simulink model "System_Modell"  (R2017b)
settings: Solver=VariableStepAuto  StartTime=0.0  StopTime=10  RelTol=1e-3
settings Model: Creator=张紫薇  LastModifiedBy=张紫薇

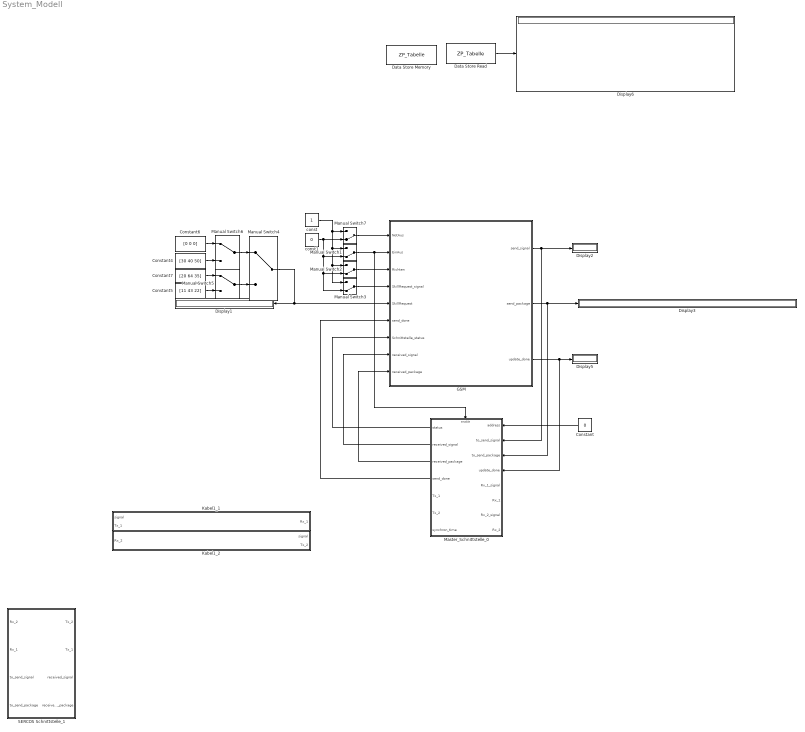
== system System_Modell ==
  Constant : Constant  Value=0
  Constant4 : Constant  Value=[30 40 50]
  Constant5 : Constant  Value=[11 43 22]
  Constant6 : Constant  Value=[0 0 0]
  Constant7 : Constant  Value=[20 64 35]
  Data Store Memory : DataStoreMemory  DataStoreName=ZP_Tabelle  ReadBeforeWriteMsg=warning  WriteAfterWriteMsg=warning  WriteAfterReadMsg=warning  InitialValue=zeros(10,7)  ShowAdditionalParam=off  OutDataTypeStr=double  Dimensions=[10 7]
  Data Store Read : DataStoreRead  DataStoreName=ZP_Tabelle
  Display{1..3,5..6} (5 alike) : Display
  "GSM " : Subsystem
  Kabel1_1 : Subsystem
  Kabel1_2 : Subsystem
  Manual Switch{1..3,7} (4 alike) : ManualSwitch  CurrentSetting=0
  Manual Switch4 : ManualSwitch
  Manual Switch5 : ManualSwitch
  Manual Switch6 : ManualSwitch
  Master_Schnittstelle_0 : Subsystem
  SERCOS Schnittstelle_1 : Subsystem
  const : Constant  OutDataTypeStr=boolean
  const1 : Constant  Value=0  OutDataTypeStr=boolean
  wires:
  Manual Switch6/1 -> Manual Switch4/1
  Constant5/1 -> Manual Switch5/2
  Manual Switch5/1 -> Manual Switch4/2
  Manual Switch3/1 -> "GSM "/4(SkillRequest_signal)
  Data Store Read/1 -> Display6/1
  Constant7/1 -> Manual Switch5/1
  const1/1 -> Manual Switch2/2, Manual Switch3/2, Manual Switch1/2, Manual Switch7/2
  "GSM "/2(send_package) -> Display3/1, Master_Schnittstelle_0/3(to_send_package)
  "GSM "/3(update_done) -> Master_Schnittstelle_0/4(update_done), Display5/1
  const/1 -> Manual Switch3/1, Manual Switch2/1, Manual Switch1/1, Manual Switch7/1
  Manual Switch7/1 -> "GSM "/1(NotAus)
  Constant6/1 -> Manual Switch6/1
  Manual Switch2/1 -> "GSM "/3(Richten)
  Manual Switch1/1 -> Master_Schnittstelle_0/Enable, "GSM "/2(EinAus)
  Manual Switch4/1 -> "GSM "/5(SkillRequest), Display1/1
  "GSM "/1(send_signal) -> Display2/1, Master_Schnittstelle_0/2(to_send_signal)
  Constant4/1 -> Manual Switch6/2
  Master_Schnittstelle_0/1(status) -> "GSM "/7(Schnittstelle_status)
  Master_Schnittstelle_0/4(send_done) -> "GSM "/6(send_done)
  Master_Schnittstelle_0/2(received_signal) -> "GSM "/8(received_signal)
  Master_Schnittstelle_0/3(received_package) -> "GSM "/9(received_package)
  Constant/1 -> Master_Schnittstelle_0/1(address)

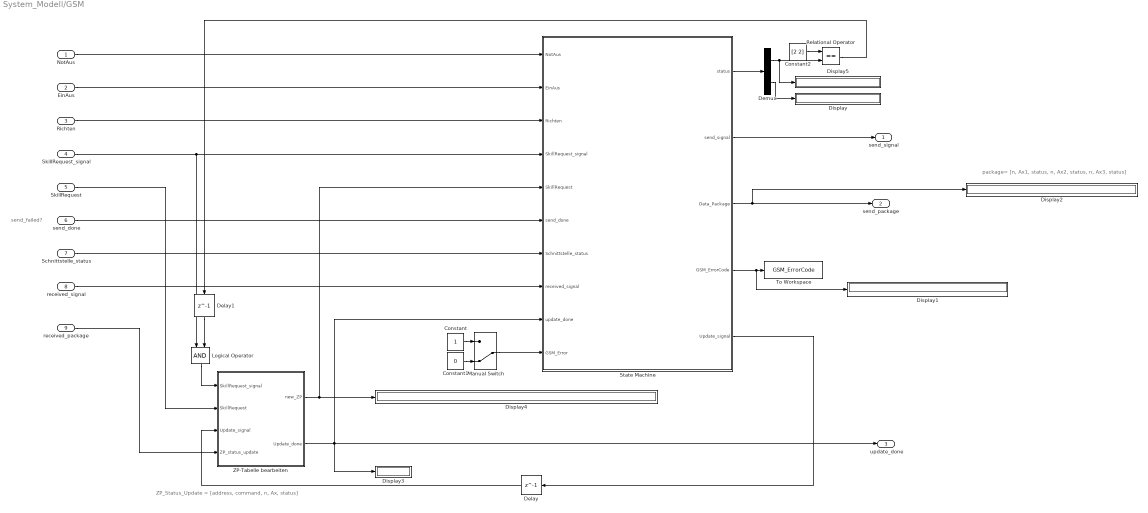
== system System_Modell/GSM  ==
  note: send_failed?
  note: package= [n, Ax1, status, n, Ax2, status, n, Ax3, status]
  note: ZP_Status_Update = [address, command, n, Ax, status]
  NotAus : Inport  OutDataTypeStr=boolean
  EinAus : Inport  Port=2  OutDataTypeStr=boolean
  Richten : Inport  Port=3  OutDataTypeStr=boolean
  SkillRequest_signal : Inport  Port=4  OutDataTypeStr=boolean
  SkillRequest : Inport  Port=5  OutDataTypeStr=double  PortDimensions=3
  send_done : Inport  Port=6  OutDataTypeStr=boolean
  Schnittstelle_status : Inport  Port=7  OutDataTypeStr=double
  received_signal : Inport  Port=8  OutDataTypeStr=boolean
  received_package : Inport  Port=9  OutDataTypeStr=double  PortDimensions=5
  Constant : Constant  OutDataTypeStr=boolean
  Constant1 : Constant  Value=0  OutDataTypeStr=boolean
  Constant2 : Constant  Value=[2 2]  OutDataTypeStr=double
  Delay : Delay  DelayLength=1
  Delay1 : Delay  DelayLength=1
  Demux : Demux  Outputs=2
  Display{,1..5} (6 alike) : Display
  Logical Operator : Logic  AllPortsSameDT=off  OutDataTypeStr=boolean
  Manual Switch : ManualSwitch  CurrentSetting=0
  Relational Operator : RelationalOperator  Operator===  OutDataTypeStr=boolean  RndMeth=Simplest
  State Machine : Stateflow chart  TreatAsAtomicUnit=on
  To Workspace : ToWorkspace  VariableName=GSM_ErrorCode  SaveFormat=Timeseries  SampleTime=-1
  ZP-Tabelle bearbeiten : Subsystem
  send_signal : Outport  OutDataTypeStr=boolean
  send_package : Outport  Port=2  OutDataTypeStr=double  PortDimensions=7
  update_done : Outport  Port=3
  wires:
  received_signal/1 -> State Machine/8(received_signal)
  Richten/1 -> State Machine/3(Richten)
  NotAus/1 -> State Machine/1(NotAus)
  EinAus/1 -> State Machine/2(EinAus)
  Schnittstelle_status/1 -> State Machine/7(Schnittstelle_status)
  State Machine/4(GSM_ErrorCode) -> Display1/1, To Workspace/1
  SkillRequest_signal/1 -> State Machine/4(SkillRequest_signal), Logical Operator/1
  SkillRequest/1 -> ZP-Tabelle bearbeiten/2(SkillRequest)
  Constant/1 -> Manual Switch/1
  Constant1/1 -> Manual Switch/2
  Manual Switch/1 -> State Machine/10(GSM_Error)
  State Machine/2(send_signal) -> send_signal/1
  State Machine/3(Data_Package) -> Display2/1, send_package/1
  received_package/1 -> ZP-Tabelle bearbeiten/4(ZP_status_update)
  ZP-Tabelle bearbeiten/1(new_ZP) -> State Machine/5(SkillRequest), Display4/1
  send_done/1 -> State Machine/6(send_done)
  ZP-Tabelle bearbeiten/2(Update_done) -> update_done/1, State Machine/9(update_done), Display3/1
  State Machine/5(Update_signal) -> Delay/1
  Delay/1 -> ZP-Tabelle bearbeiten/3(Update_signal)
  Demux/2 -> Display/1
  State Machine/1(status) -> Demux/1
  Constant2/1 -> Relational Operator/1
  Demux/1 -> Display5/1, Relational Operator/2
  Relational Operator/1 -> Delay1/1
  Delay1/1 -> Logical Operator/2
  Logical Operator/1 -> ZP-Tabelle bearbeiten/1(SkillRequest_signal)

== system System_Modell/Kabel1_1 ==
  Rx_1 : Inport
  Delay : Delay  DelayLength=1
  signal : Outport
  Tx_1 : Outport  Port=2
  wires:
  Rx_1/1 -> Delay/1, Tx_1/1
  Delay/1 -> signal/1

== system System_Modell/Kabel1_2 ==
  Rx_2 : Inport
  Delay : Delay  DelayLength=1
  signal : Outport
  Tx_2 : Outport  Port=2
  wires:
  Rx_2/1 -> Delay/1, Tx_2/1
  Delay/1 -> signal/1

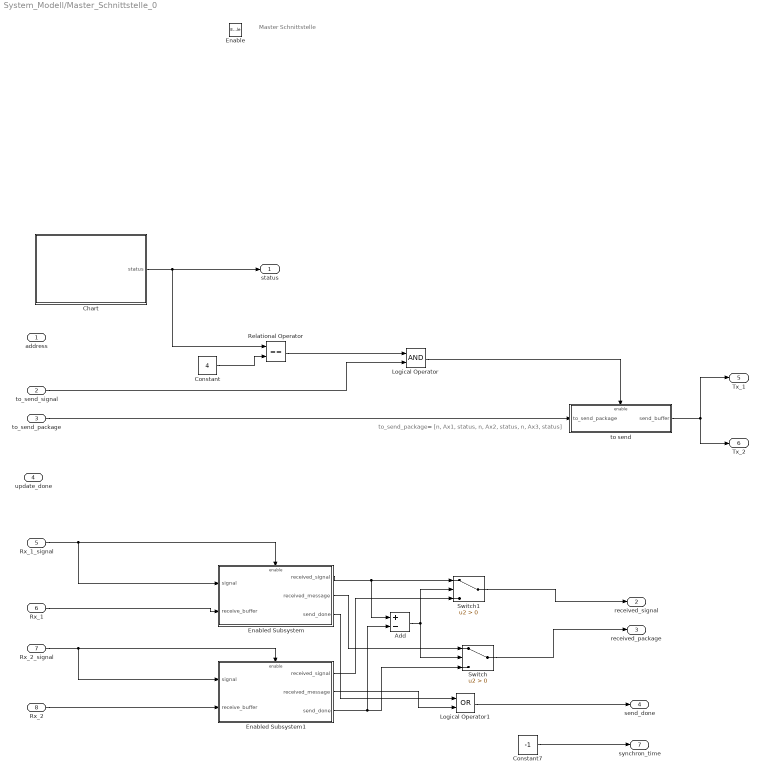
== system System_Modell/Master_Schnittstelle_0 ==
  note: Master Schnittstelle
  note: to_send_package= [n, Ax1, status, n, Ax2, status, n, Ax3, status]
  address : Inport
  to_send_signal : Inport  Port=2
  to_send_package : Inport  Port=3
  update_done : Inport  Port=4
  Rx_1_signal : Inport  Port=5
  Rx_1 : Inport  Port=6
  Rx_2_signal : Inport  Port=7
  Rx_2 : Inport  Port=8
  Enable : EnablePort
  Add : Sum  Inputs=+-
  Chart : Stateflow chart  TreatAsAtomicUnit=on
  Constant : Constant  Value=4
  Constant7 : Constant  Value=-1
  Enabled Subsystem : Subsystem  TreatAsAtomicUnit=on
  Enabled Subsystem1 : Subsystem  TreatAsAtomicUnit=on
  Logical Operator : Logic  AllPortsSameDT=off  OutDataTypeStr=boolean
  Logical Operator1 : Logic  Operator=OR  AllPortsSameDT=off  OutDataTypeStr=boolean
  Relational Operator : RelationalOperator  Operator===  OutDataTypeStr=boolean  RndMeth=Simplest
  Switch : Switch  Criteria=u2 > Threshold
  Switch1 : Switch  Criteria=u2 > Threshold
  to send : Subsystem  TreatAsAtomicUnit=on
  status : Outport
  received_signal : Outport  Port=2
  received_package : Outport  Port=3
  send_done : Outport  Port=4
  Tx_1 : Outport  Port=5
  Tx_2 : Outport  Port=6
  synchron_time : Outport  Port=7
  wires:
  Constant/1 -> Relational Operator/2
  Relational Operator/1 -> Logical Operator/1
  to_send_signal/1 -> Logical Operator/2
  Logical Operator/1 -> to send/Enable
  to_send_package/1 -> to send/1(to_send_package)
  Rx_1/1 -> Enabled Subsystem/2(receive_buffer)
  Chart/1(status) -> status/1, Relational Operator/1
  Rx_1_signal/1 -> Enabled Subsystem/Enable, Enabled Subsystem/1(signal)
  Rx_2_signal/1 -> Enabled Subsystem1/Enable, Enabled Subsystem1/1(signal)
  Rx_2/1 -> Enabled Subsystem1/2(receive_buffer)
  Enabled Subsystem/2(received_message) -> Switch/1
  Enabled Subsystem1/3(send_done) -> Add/2, Switch/3
  Switch/1 -> received_package/1
  Enabled Subsystem/1(received_signal) -> Add/1, Switch1/1
  Enabled Subsystem1/1(received_signal) -> Switch1/3
  Switch1/1 -> received_signal/1
  Add/1 -> Switch1/2, Switch/2
  to send/1(send_buffer) -> Tx_2/1, Tx_1/1
  Enabled Subsystem/3(send_done) -> Logical Operator1/1
  Enabled Subsystem1/2(received_message) -> Logical Operator1/2
  Logical Operator1/1 -> send_done/1
  Constant7/1 -> synchron_time/1

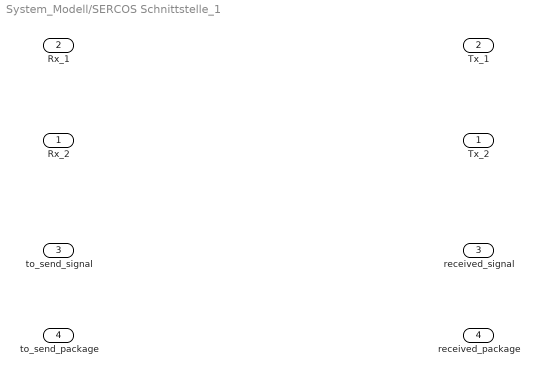
== system System_Modell/SERCOS Schnittstelle_1 ==
  Rx_2 : Inport
  Rx_1 : Inport  Port=2
  to_send_signal : Inport  Port=3
  to_send_package : Inport  Port=4
  Tx_2 : Outport
  Tx_1 : Outport  Port=2
  received_signal : Outport  Port=3
  received_package : Outport  Port=4

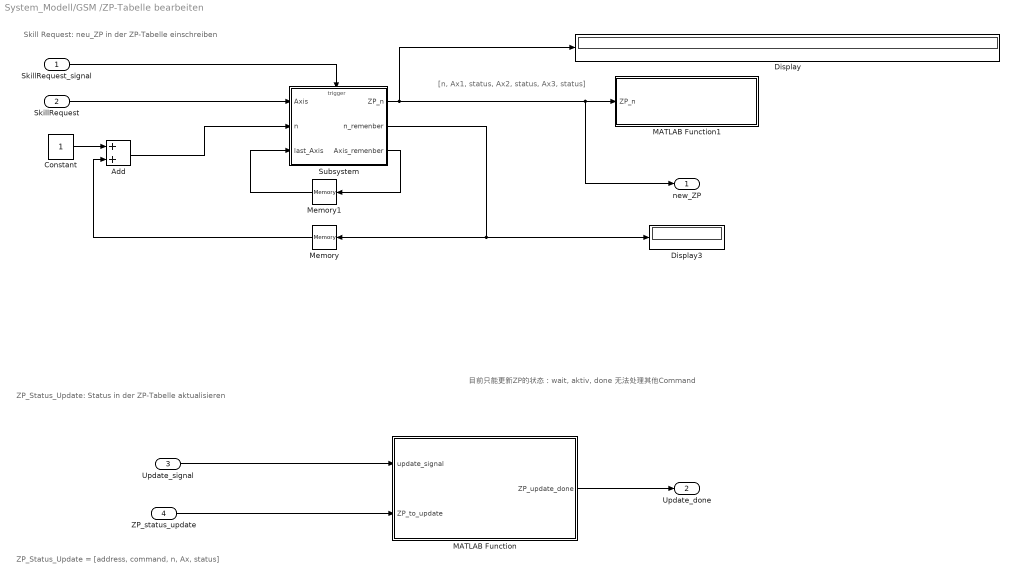
== system System_Modell/GSM /ZP-Tabelle bearbeiten ==
  note: ZP_Status_Update = [address, command, n, Ax, status]
  note: Skill Request: neu_ZP in der ZP-Tabelle einschreiben
  note: ZP_Status_Update: Status in der ZP-Tabelle aktualisieren
  note: [n, Ax1, status, Ax2, status, Ax3, status]
  note: 目前只能更新ZP的状态：wait, aktiv, done
      | 无法处理其他Command
  SkillRequest_signal : Inport  OutDataTypeStr=boolean
  SkillRequest : Inport  Port=2  OutDataTypeStr=double  PortDimensions=3
  Update_signal : Inport  Port=3  OutDataTypeStr=boolean
  ZP_status_update : Inport  Port=4  OutDataTypeStr=double  PortDimensions=5
  Add : Sum
  Constant : Constant
  Display : Display
  Display3 : Display
  MATLAB Function : MATLAB Function  TreatAsAtomicUnit=on
  MATLAB Function1 : MATLAB Function  TreatAsAtomicUnit=on
  Memory : Memory
  Memory1 : Memory  InitialCondition=[0 0 0]
  Subsystem : Subsystem
  new_ZP : Outport
  Update_done : Outport  Port=2  OutDataTypeStr=boolean
  wires:
  Memory1/1 -> Subsystem/3(last_Axis)
  Subsystem/3(Axis_remenber) -> Memory1/1
  SkillRequest/1 -> Subsystem/1(Axis)
  Update_signal/1 -> MATLAB Function/1(update_signal)
  Add/1 -> Subsystem/2(n)
  ZP_status_update/1 -> MATLAB Function/2(ZP_to_update)
  MATLAB Function/1(ZP_update_done) -> Update_done/1
  Constant/1 -> Add/1
  SkillRequest_signal/1 -> Subsystem/Trigger
  Memory/1 -> Add/2
  Subsystem/2(n_remenber) -> Memory/1, Display3/1
  Subsystem/1(ZP_n) -> Display/1, MATLAB Function1/1(ZP_n), new_ZP/1

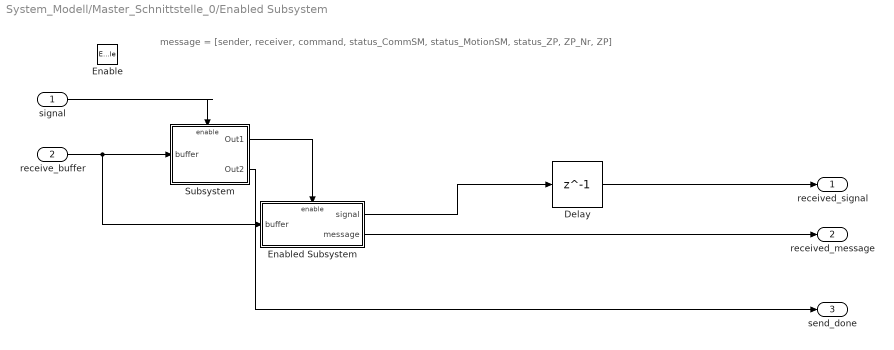
== system System_Modell/Master_Schnittstelle_0/Enabled Subsystem ==
  note: message = [sender, receiver, command, status_CommSM, status_MotionSM, status_ZP, ZP_Nr, ZP]
  signal : Inport
  receive_buffer : Inport  Port=2
  Enable : EnablePort
  Delay : Delay  DelayLength=1
  Enabled Subsystem : Subsystem  TreatAsAtomicUnit=on
  Subsystem : Subsystem
  received_signal : Outport
  received_message : Outport  Port=2
  send_done : Outport  Port=3
  wires:
  receive_buffer/1 -> Enabled Subsystem/1(buffer), Subsystem/1(buffer)
  Subsystem/1(Out1) -> Enabled Subsystem/Enable
  signal/1 -> Subsystem/Enable
  Enabled Subsystem/2(message) -> received_message/1
  Enabled Subsystem/1(signal) -> Delay/1
  Delay/1 -> received_signal/1
  Subsystem/2(Out2) -> send_done/1

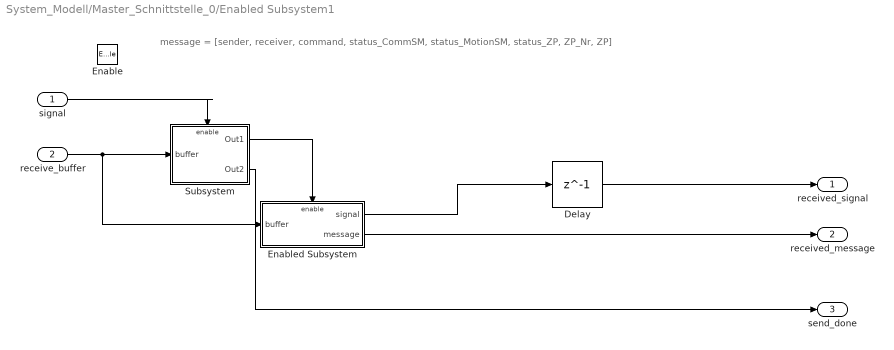
== system System_Modell/Master_Schnittstelle_0/Enabled Subsystem1 ==
  note: message = [sender, receiver, command, status_CommSM, status_MotionSM, status_ZP, ZP_Nr, ZP]
  signal : Inport
  receive_buffer : Inport  Port=2
  Enable : EnablePort
  Delay : Delay  DelayLength=1
  Enabled Subsystem : Subsystem  TreatAsAtomicUnit=on
  Subsystem : Subsystem
  received_signal : Outport
  received_message : Outport  Port=2
  send_done : Outport  Port=3
  wires:
  receive_buffer/1 -> Enabled Subsystem/1(buffer), Subsystem/1(buffer)
  Subsystem/1(Out1) -> Enabled Subsystem/Enable
  signal/1 -> Subsystem/Enable
  Enabled Subsystem/2(message) -> received_message/1
  Enabled Subsystem/1(signal) -> Delay/1
  Delay/1 -> received_signal/1
  Subsystem/2(Out2) -> send_done/1

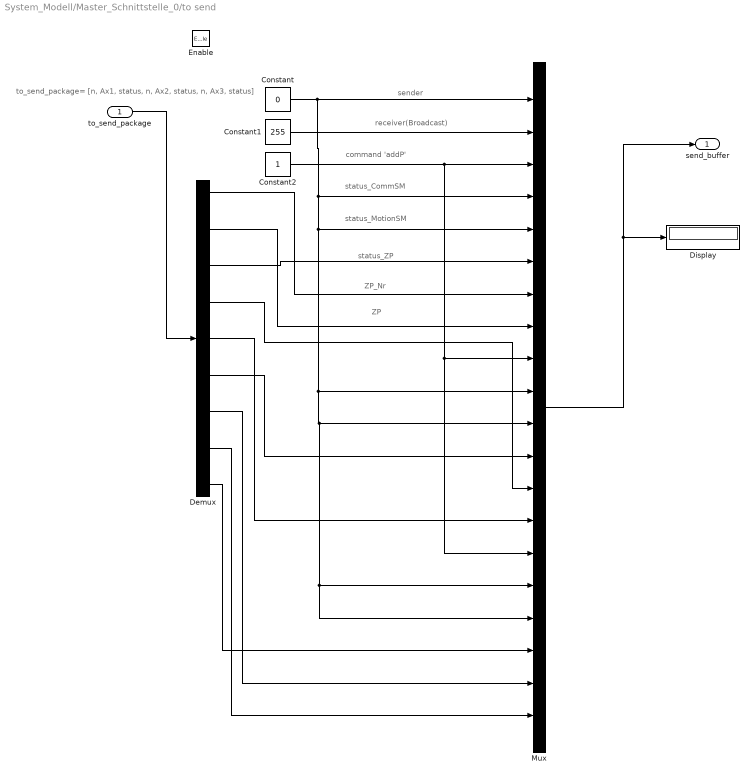
== system System_Modell/Master_Schnittstelle_0/to send ==
  note: ZP
  note: ZP_Nr
  note: status_ZP
  note: status_MotionSM
  note: status_CommSM
  note: command 'addP'
  note: receiver(Broadcast)
  note: sender
  note: to_send_package= [n, Ax1, status, n, Ax2, status, n, Ax3, status]
  to_send_package : Inport
  Enable : EnablePort
  Constant : Constant  Value=0
  Constant1 : Constant  Value=255
  Constant2 : Constant
  Demux : Demux  Outputs=9
  Display : Display
  Mux : Mux  Inputs=20
  send_buffer : Outport
  wires:
  to_send_package/1 -> Demux/1
  Constant/1 -> Mux/1, Mux/5, Mux/10, Mux/16, Mux/17, Mux/11, Mux/4
  Constant1/1 -> Mux/2
  Constant2/1 -> Mux/15, Mux/9, Mux/3
  Demux/3 -> Mux/6
  Demux/1 -> Mux/7
  Demux/2 -> Mux/8
  Demux/6 -> Mux/12
  Demux/4 -> Mux/13
  Demux/5 -> Mux/14
  Demux/9 -> Mux/18
  Demux/7 -> Mux/19
  Demux/8 -> Mux/20
  Mux/1 -> Display/1, send_buffer/1

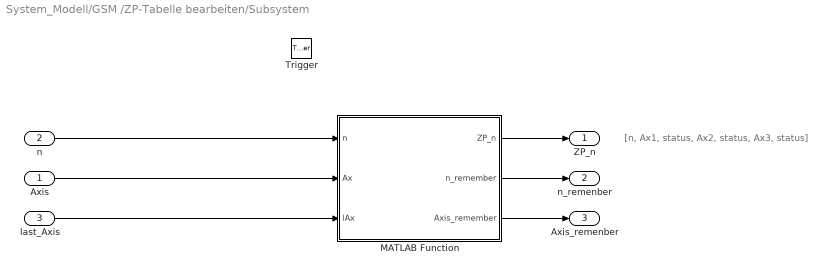
== system System_Modell/GSM /ZP-Tabelle bearbeiten/Subsystem ==
  note: [n, Ax1, status, Ax2, status, Ax3, status]
  Axis : Inport
  n : Inport  Port=2
  last_Axis : Inport  Port=3
  Trigger : TriggerPort  VariantControl=Variant  PortDimensions=1
  MATLAB Function : MATLAB Function  TreatAsAtomicUnit=on
  ZP_n : Outport
  n_remenber : Outport  Port=2
  Axis_remenber : Outport  Port=3
  wires:
  n/1 -> MATLAB Function/1(n)
  Axis/1 -> MATLAB Function/2(Ax)
  MATLAB Function/1(ZP_n) -> ZP_n/1
  last_Axis/1 -> MATLAB Function/3(lAx)
  MATLAB Function/2(n_remember) -> n_remenber/1
  MATLAB Function/3(Axis_remember) -> Axis_remenber/1

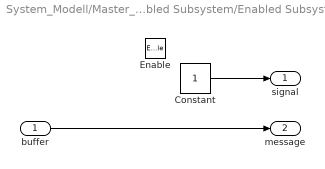
== system System_Modell/Master_Schnittstelle_0/Enabled Subsystem/Enabled Subsystem ==
  buffer : Inport
  Enable : EnablePort
  Constant : Constant
  signal : Outport
  message : Outport  Port=2
  wires:
  buffer/1 -> message/1
  Constant/1 -> signal/1

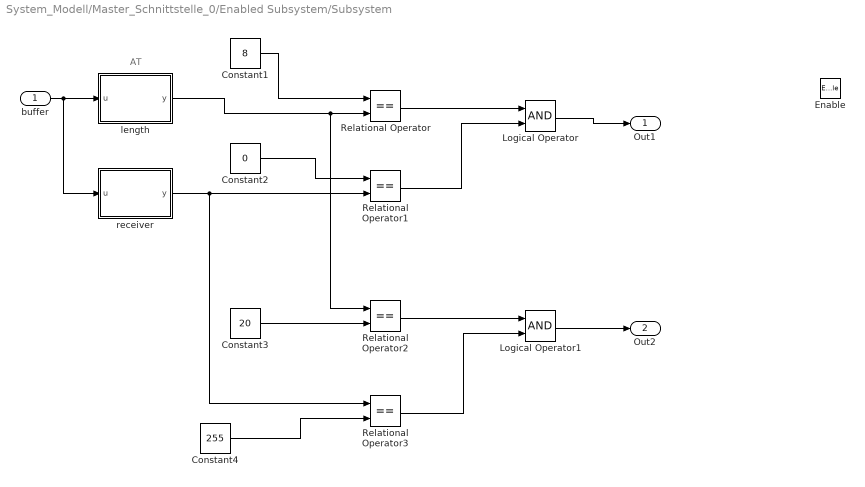
== system System_Modell/Master_Schnittstelle_0/Enabled Subsystem/Subsystem ==
  note: AT
  buffer : Inport
  Enable : EnablePort
  Constant1 : Constant  Value=8
  Constant2 : Constant  Value=0
  Constant3 : Constant  Value=20
  Constant4 : Constant  Value=255
  Logical Operator : Logic  AllPortsSameDT=off  OutDataTypeStr=boolean
  Logical Operator1 : Logic  AllPortsSameDT=off  OutDataTypeStr=boolean
  Relational Operator{,1..3} (4 alike) : RelationalOperator  Operator===  OutDataTypeStr=boolean  RndMeth=Simplest
  length : MATLAB Function  TreatAsAtomicUnit=on
  receiver : MATLAB Function  TreatAsAtomicUnit=on
  Out1 : Outport
  Out2 : Outport  Port=2
  wires:
  Constant2/1 -> Relational Operator1/1
  buffer/1 -> receiver/1(u), length/1(u)
  length/1(y) -> Relational Operator2/1, Relational Operator/2
  Constant1/1 -> Relational Operator/1
  receiver/1(y) -> Relational Operator3/1, Relational Operator1/2
  Relational Operator/1 -> Logical Operator/1
  Relational Operator1/1 -> Logical Operator/2
  Logical Operator/1 -> Out1/1
  Constant3/1 -> Relational Operator2/2
  Relational Operator2/1 -> Logical Operator1/1
  Constant4/1 -> Relational Operator3/2
  Relational Operator3/1 -> Logical Operator1/2
  Logical Operator1/1 -> Out2/1

== system System_Modell/Master_Schnittstelle_0/Enabled Subsystem1/Enabled Subsystem ==
  buffer : Inport
  Enable : EnablePort
  Constant : Constant
  signal : Outport
  message : Outport  Port=2
  wires:
  buffer/1 -> message/1
  Constant/1 -> signal/1

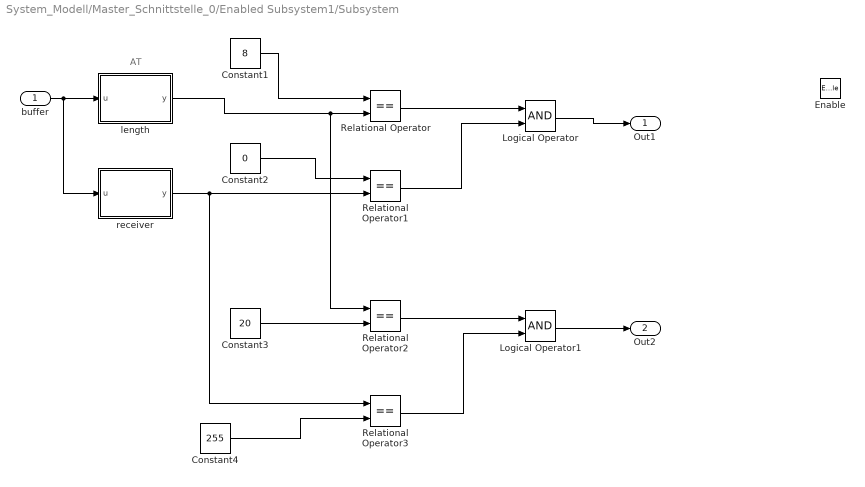
== system System_Modell/Master_Schnittstelle_0/Enabled Subsystem1/Subsystem ==
  note: AT
  buffer : Inport
  Enable : EnablePort
  Constant1 : Constant  Value=8
  Constant2 : Constant  Value=0
  Constant3 : Constant  Value=20
  Constant4 : Constant  Value=255
  Logical Operator : Logic  AllPortsSameDT=off  OutDataTypeStr=boolean
  Logical Operator1 : Logic  AllPortsSameDT=off  OutDataTypeStr=boolean
  Relational Operator{,1..3} (4 alike) : RelationalOperator  Operator===  OutDataTypeStr=boolean  RndMeth=Simplest
  length : MATLAB Function  TreatAsAtomicUnit=on
  receiver : MATLAB Function  TreatAsAtomicUnit=on
  Out1 : Outport
  Out2 : Outport  Port=2
  wires:
  Constant2/1 -> Relational Operator1/1
  buffer/1 -> receiver/1(u), length/1(u)
  length/1(y) -> Relational Operator2/1, Relational Operator/2
  Constant1/1 -> Relational Operator/1
  receiver/1(y) -> Relational Operator3/1, Relational Operator1/2
  Relational Operator/1 -> Logical Operator/1
  Relational Operator1/1 -> Logical Operator/2
  Logical Operator/1 -> Out1/1
  Constant3/1 -> Relational Operator2/2
  Relational Operator2/1 -> Logical Operator1/1
  Constant4/1 -> Relational Operator3/2
  Relational Operator3/1 -> Logical Operator1/2
  Logical Operator1/1 -> Out2/1

== stateflow chart System_Modell/GSM /State Machine ==
  settings: executeAtInitialization=1
  state NotAus
    entry: status=[1 0 0 0]
  state Aus
    entry: status=[0 0 0 0]
  state Ein
    entry: status=[2 0 0 0]
    note: status_Schnittstelle: CP0 - CP4
    state Init
      entry: status=[2 1 0 0]
    state Error
      entry: status=[2 3 0 0];
    state Run
      entry: status= [2 2 0 0]
      state Stand_By
        entry: status = [2 2 1 0];
      state Send_ZP
        entry: status = [2 2 2 0]; send_signal=SkillRequest_signal; Data_Package = SkillRequest
      note: wann send_signal=0 ???
      state ZP_Status_Update
        entry: status = [2 2 3 0]; Update_signal = received_signal
      note: ZP_Status_Update = [address, command, n, Ax, status]
      note: received_package = [address, command, n, Ax, status]
      (default) -> Stand_By
      Stand_By -> Send_ZP [order 1] : [SkillRequest_signal && ~send_done]
      Send_ZP -> Stand_By : [send_done && ~SkillRequest_signal]{send_signal=false;}
      ZP_Status_Update -> Stand_By : [update_done && ~received_signal]{Update_signal=false;}
      Stand_By -> ZP_Status_Update [order 2] : [received_signal && ~update_done]
    Error -> Init : [GSM_Error==0] {GSM_ErrorCode=[0 0  0 0]}
    (default) -> Init
    Init -> Error [order 2] : [GSM_Error]{GSM_ErrorCode=status}
    Run -> Error [order 1] : [GSM_Error]{GSM_ErrorCode=status}
    Run -> Init [order 2] : [Schnittstelle_status~=4 && GSM_Error==0]
    Init -> Run [order 1] : [Schnittstelle_status==4]
  NotAus -> Aus [order 2] : [EinAus==0]
  Aus -> NotAus [order 1] : [EinAus==1 && NotAus==1]
  (default) -> Aus
  Ein -> NotAus [order 2] : [NotAus==1]
  NotAus -> Ein [order 1] : [NotAus==0 && Richten==1]
  Ein -> Aus [order 1] : [EinAus==0]
  Aus -> Ein [order 2] : [EinAus==1 && NotAus==0]
  data: NotAus input boolean; EinAus input boolean; Richten input boolean; SkillRequest_signal input boolean; SkillRequest input double size=7; send_done input boolean; Schnittstelle_status input double; status output double; send_signal output boolean; received_signal input boolean; update_done input boolean; GSM_Error input boolean; Data_Package output double size=7; GSM_ErrorCode output double; Update_signal output boolean size=1

== matlab function System_Modell/GSM /ZP-Tabelle bearbeiten/MATLAB Function ==
  data: update_signal input boolean; ZP_to_update input double size=5; ZP_update_done output boolean; ZP_Tabelle data_store_memory
%ZP_Status_Update = [address, command, n, Ax, status]
%function [ZP_update_done, Update_Data] = Status_Update(update_signal, ZP_to_update, ZP_Tab)

function ZP_update_done  = Status_Update(update_signal, ZP_to_update)

global ZP_Tabelle

N=0;
m=0;
n=0;

if update_signal == true
    address = ZP_to_update(1);
    m = 2 * address + 1;
    n = ZP_to_update(3);
    status = ZP_to_update(5);
    
    for i=1:10
        if ZP_Tabelle(i,1) == n
            N = i;              %ZP_N bestimmen
            break
        end
    end
    
    %N==1, status aktualisieren
    %N>1 && (status von ZP_N-1 == 'done'), status aktualisieren
    if (N == 1) || (N>1 && (ZP_Tabelle(N-1,3) == ZP_Tabelle(N-1,5) == ZP_Tabelle(N-1,7) == 3))
        ZP_Tabelle(N,m) = status;
        ZP_update_done = true;
    else        
        ZP_update_done = false;
    end
else
    ZP_update_done = false;
end

%Update_Data = ZP_Tabelle;

== stateflow chart System_Modell/Master_Schnittstelle_0/Chart ==
  state Start
    entry: status=-2
  state CP1
    entry: status=1
  state NRT
    entry: status=-1
  state CP0
    entry: status=0
  state CP2
    entry: status=2
  state CP3
    entry: status=3
  state CP4
    entry: status=4
  (default) -> Start
  CP0 -> CP1 [order 1]
  CP1 -> CP0 [order 2]
  Start -> NRT
  CP1 -> CP2 [order 1]
  CP2 -> CP0 [order 2]
  NRT -> CP0
  CP0 -> NRT [order 2]
  CP2 -> CP3 [order 1]
  CP4 -> CP0
  CP3 -> CP0 [order 2]
  CP3 -> CP4 [order 1]
  data: status output

== matlab function System_Modell/Master_Schnittstelle_0/Enabled Subsystem/Subsystem/length ==
  data: u input; y output
function y = fcn(u)

y = length(u);

== matlab function System_Modell/Master_Schnittstelle_0/Enabled Subsystem/Subsystem/receiver ==
  data: u input; y output
function y = fcn(u)

y = u(2);

== matlab function System_Modell/Master_Schnittstelle_0/Enabled Subsystem1/Subsystem/length ==
  data: u input; y output
function y = fcn(u)

y = length(u);

== matlab function System_Modell/Master_Schnittstelle_0/Enabled Subsystem1/Subsystem/receiver ==
  data: u input; y output
function y = fcn(u)

y = u(2);

== matlab function System_Modell/GSM /ZP-Tabelle bearbeiten/MATLAB Function1 ==
  data: ZP_n input; ZP_Tabelle data_store_memory
%ZP_n = [n, Ax1, status1, Ax2, status2, Ax3, status3];
%function ZP_newTable = new_ZP(ZP_n)

function new_ZP(ZP_n)

global ZP_Tabelle

m=0;
n = ZP_n(1);

for i = 1:10
    if ZP_Tabelle(i,1) == n
        break;
    end
    if ZP_Tabelle(i,1) == 0
        m=i;
        break
    end
end

if m ~= 0
    ZP_Tabelle(m,:) = ZP_n;
end

end

== matlab function System_Modell/GSM /ZP-Tabelle bearbeiten/Subsystem/MATLAB Function ==
  data: n input; ZP_n output double size=[1 7]; Ax input; lAx input; n_remember output; Axis_remember output
%ZP_n = [n, Ax1, status, Ax2, status, Ax3, status];

function [ZP_n, n_remember, Axis_remember] = Zielposition(n, Ax, lAx)

if ((Ax(1) == lAx(1)) && (Ax(2) == lAx(2)) && (Ax(3) == lAx(3))) == 0   %wiederholte Position filtern
    ZP_n = [n, Ax(1), 1, Ax(2), 1, Ax(3), 1];
    n_remember = n;
else
    ZP_n = [n-1, lAx(1), 1, lAx(2), 1, lAx(3),1];     %ZP_n ändert sich nicht
    n_remember = n-1;
end

Axis_remember = Ax;
end
